simulink model "RW_1"  (R2018a)
settings: Solver=ode4  StartTime=0  StopTime=25000  FixedStep=ConfParam.confOrbit.dt  RelTol=1e-3
undefined symbols (not defined in the file): ConfParam
libraries: sharedtransform x2, Command x1, Date x1, KepOrbit x1, Estimator x1, BdotController x1, RWS_PDcontroller x1, IGRF x1, SunEphemeris_MathWorks x1, MTB x1, Magnetometer x1, AeroTorqueA x1
settings Model: Creator=Cédric  LastModifiedBy=Cédric
settings DataIOCC: SaveTime=off
settings DebuggingCC: MultiTaskRateTransMsg=warning

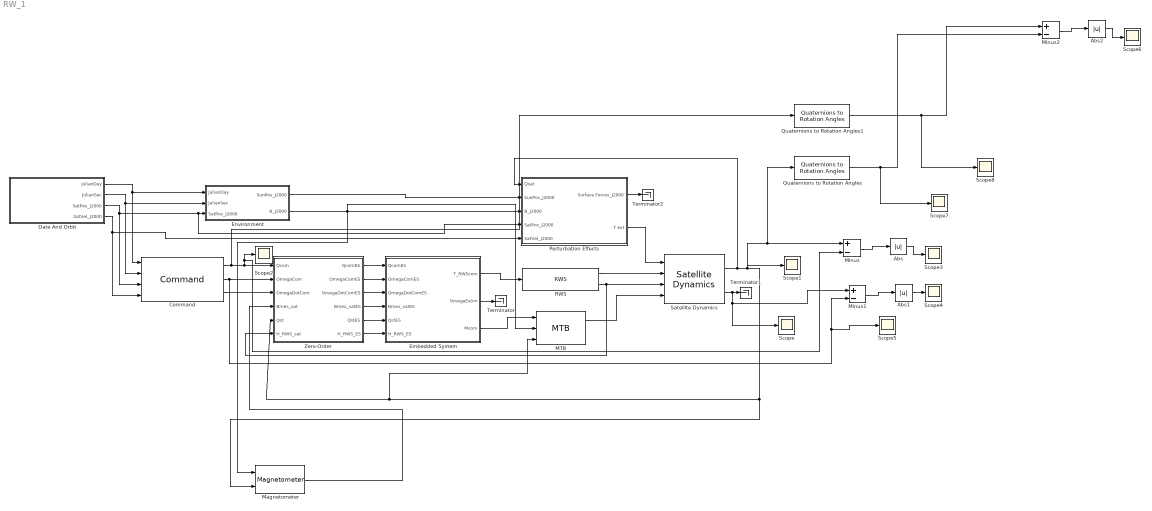
== system RW_1 ==
  Abs : Abs
  Abs1 : Abs
  Abs2 : Abs
  Command : Command/Command
  Date And Orbit : Subsystem
  Embedded System : Subsystem
  Environment : Subsystem
  MTB : MTB/MTB
  Magnetometer : Magnetometer/Magnetometer
  Minus : Sum  Inputs=+-
  Minus1 : Sum  Inputs=+-
  Minus2 : Sum  Inputs=+-
  Perturbation Effects : Subsystem
  Quaternions to Rotation Angles : sharedtransform/Quaternions to Rotation Angles  rotationOrder=ZYX  aMode=aMode
      settings: SourceProductBaseCode=AE
  Quaternions to Rotation Angles1 : sharedtransform/Quaternions to Rotation Angles  rotationOrder=ZYX  aMode=aMode
      settings: SourceProductBaseCode=AE
  RWS : RWS/RWS
  Satellite Dynamics : SatDyn/Satellite Dynamics
  Scope{,1..8} (9 alike) : Scope
  Terminator : Terminator
  Terminator1 : Terminator
  Terminator2 : Terminator
  Zero-Order : Subsystem
  wires:
  Date And Orbit/1(JulianDay) -> Environment/1(JulianDay), Command/1
  Date And Orbit/2(JulianSec) -> Environment/2(JulianSec), Command/2
  Date And Orbit/3(SatPos_J2000) -> Perturbation Effects/4(SatPos_J2000), Environment/3(SatPos_J2000), Command/3
  Date And Orbit/4(SatVel_J2000) -> Perturbation Effects/5(SatVel_J2000), Command/4
  Environment/1(SunPos_J2000) -> Perturbation Effects/2(SunPos_J2000)
  Environment/2(B_J2000) -> Perturbation Effects/3(B_J2000), Magnetometer/1, MTB/2
  Command/1 -> Quaternions to Rotation Angles1/1, Minus/2, Scope2/1, Zero-Order/1(Qcom)
  Command/2 -> Scope5/1, Minus1/2, Zero-Order/2(OmegaCom)
  Command/3 -> Zero-Order/3(OmegaDotCom)
  Zero-Order/1(QcomES) -> Embedded System/1(QcomES)
  Zero-Order/2(OmegaComES) -> Embedded System/2(OmegaComES)
  Zero-Order/3(OmegaDotComES) -> Embedded System/3(OmegaDotComES)
  Zero-Order/4(Bmes_satES) -> Embedded System/4(Bmes_satES)
  Zero-Order/5(QstES) -> Embedded System/5(QstES)
  Zero-Order/6(H_RWS_ES) -> Embedded System/6(H_RWS_ES)
  Embedded System/1(T_RWScom) -> RWS/1
  Embedded System/3(Mcom) -> MTB/1
  Satellite Dynamics/1 -> Perturbation Effects/1(Qsat), Scope1/1, Quaternions to Rotation Angles/1, Minus/1, MTB/3, Zero-Order/5(Qst), Magnetometer/2
  RWS/2 -> Satellite Dynamics/3, Zero-Order/6(H_RWS_sat)
  Perturbation Effects/2(T ext) -> Satellite Dynamics/1
  RWS/1 -> Satellite Dynamics/2
  MTB/1 -> Satellite Dynamics/4
  Magnetometer/1 -> Zero-Order/4(Bmes_sat)
  Embedded System/2(OmegaEstim) -> Terminator/1
  Satellite Dynamics/2 -> Minus1/1, Scope/1, Terminator1/1
  Perturbation Effects/1(Surface Forces_J2000) -> Terminator2/1
  Minus/1 -> Abs/1
  Abs/1 -> Scope3/1
  Minus1/1 -> Abs1/1
  Abs1/1 -> Scope4/1
  Abs2/1 -> Scope6/1
  Minus2/1 -> Abs2/1
  Quaternions to Rotation Angles1/1 -> Scope8/1, Minus2/1
  Quaternions to Rotation Angles/1 -> Scope7/1, Minus2/2

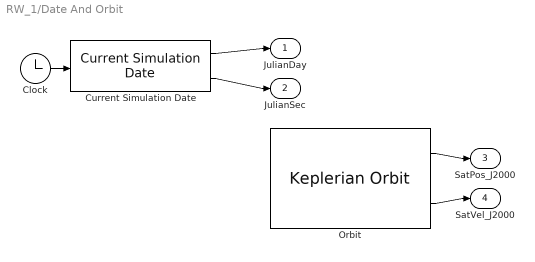
== system RW_1/Date And Orbit ==
  Clock : Clock
  Current Simulation Date : Date/Current Simulation Date
  Orbit : KepOrbit/Keplerian Orbit
  JulianDay : Outport
  JulianSec : Outport  Port=2
  SatPos_J2000 : Outport  Port=3
  SatVel_J2000 : Outport  Port=4
  wires:
  Current Simulation Date/1 -> JulianDay/1
  Current Simulation Date/2 -> JulianSec/1
  Clock/1 -> Current Simulation Date/1
  Orbit/1 -> SatPos_J2000/1
  Orbit/2 -> SatVel_J2000/1

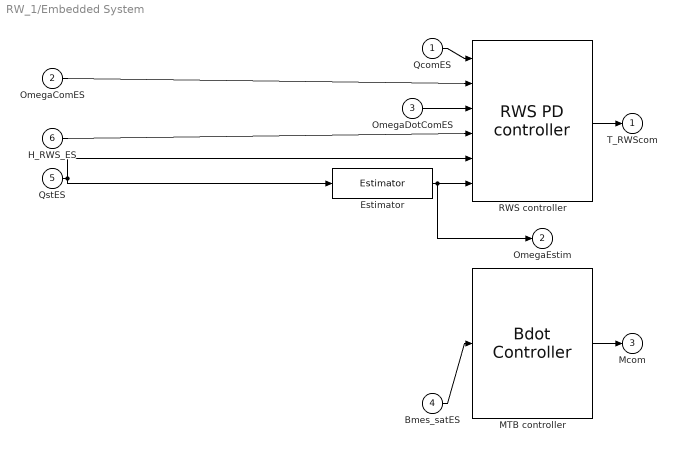
== system RW_1/Embedded System ==
  QcomES : Inport
  OmegaComES : Inport  Port=2
  OmegaDotComES : Inport  Port=3
  Bmes_satES : Inport  Port=4
  QstES : Inport  Port=5
  H_RWS_ES : Inport  Port=6
  Estimator : Estimator/Estimator
  MTB controller : BdotController/Bdot Controller
  RWS controller : RWS_PDcontroller/RWS PD controller
  T_RWScom : Outport
  OmegaEstim : Outport  Port=2
  Mcom : Outport  Port=3
  wires:
  QcomES/1 -> RWS controller/1
  OmegaComES/1 -> RWS controller/2
  OmegaDotComES/1 -> RWS controller/3
  H_RWS_ES/1 -> RWS controller/4
  QstES/1 -> RWS controller/5, Estimator/1
  Estimator/1 -> RWS controller/6, OmegaEstim/1
  RWS controller/1 -> T_RWScom/1
  Bmes_satES/1 -> MTB controller/1
  MTB controller/1 -> Mcom/1

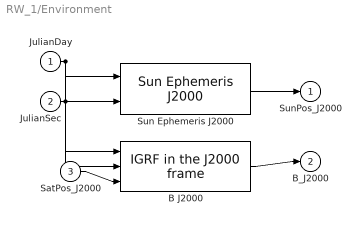
== system RW_1/Environment ==
  JulianDay : Inport
  JulianSec : Inport  Port=2
  SatPos_J2000 : Inport  Port=3
  B J2000 : IGRF/IGRF in the J2000 frame
  Sun Ephemeris J2000 : SunEphemeris_MathWorks/Sun Ephemeris J2000
  SunPos_J2000 : Outport
  B_J2000 : Outport  Port=2
  wires:
  Sun Ephemeris J2000/1 -> SunPos_J2000/1
  JulianDay/1 -> Sun Ephemeris J2000/1, B J2000/1
  JulianSec/1 -> Sun Ephemeris J2000/2, B J2000/2
  SatPos_J2000/1 -> B J2000/3
  B J2000/1 -> B_J2000/1

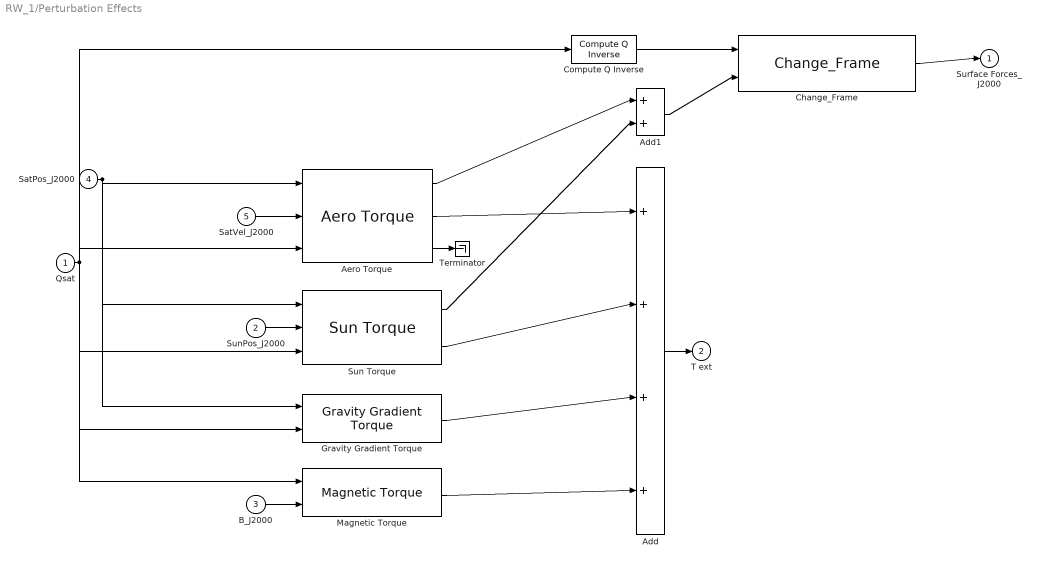
== system RW_1/Perturbation Effects ==
  Qsat : Inport
  SunPos_J2000 : Inport  Port=2
  B_J2000 : Inport  Port=3
  SatPos_J2000 : Inport  Port=4
  SatVel_J2000 : Inport  Port=5
  Add : Sum  Inputs=++++
  Add1 : Sum
  Aero Torque : AeroTorqueA/Aero Torque
  Change_Frame : ChangeFrame/Change_Frame
  Compute Q Inverse : Qinverse/Compute Q Inverse
  Gravity Gradient Torque : GravGradTorque/Gravity Gradient Torque
  Magnetic Torque : MagnTorque/Magnetic Torque
  Sun Torque : SunTorqueA/Sun Torque
  Terminator : Terminator
  Surface Forces_J2000 : Outport
  T ext : Outport  Port=2
  wires:
  Compute Q Inverse/1 -> Change_Frame/1
  Change_Frame/1 -> Surface Forces_J2000/1
  Qsat/1 -> Compute Q Inverse/1, Gravity Gradient Torque/2, Sun Torque/3, Magnetic Torque/1, Aero Torque/3
  SunPos_J2000/1 -> Sun Torque/2
  B_J2000/1 -> Magnetic Torque/2
  SatPos_J2000/1 -> Sun Torque/1, Gravity Gradient Torque/1, Aero Torque/1
  SatVel_J2000/1 -> Aero Torque/2
  Aero Torque/3 -> Terminator/1
  Add1/1 -> Change_Frame/2
  Aero Torque/1 -> Add1/1
  Sun Torque/1 -> Add1/2
  Add/1 -> T ext/1
  Aero Torque/2 -> Add/1
  Sun Torque/2 -> Add/2
  Gravity Gradient Torque/1 -> Add/3
  Magnetic Torque/1 -> Add/4

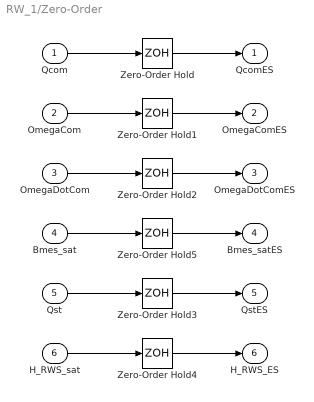
== system RW_1/Zero-Order ==
  Qcom : Inport
  OmegaCom : Inport  Port=2
  OmegaDotCom : Inport  Port=3
  Bmes_sat : Inport  Port=4
  Qst : Inport  Port=5
  H_RWS_sat : Inport  Port=6
  Zero-Order Hold{,1..5} (6 alike) : ZeroOrderHold  SampleTime=1/ConfParam.confES.frequency
  QcomES : Outport
  OmegaComES : Outport  Port=2
  OmegaDotComES : Outport  Port=3
  Bmes_satES : Outport  Port=4
  QstES : Outport  Port=5
  H_RWS_ES : Outport  Port=6
  wires:
  Qcom/1 -> Zero-Order Hold/1
  Zero-Order Hold/1 -> QcomES/1
  OmegaCom/1 -> Zero-Order Hold1/1
  Zero-Order Hold1/1 -> OmegaComES/1
  OmegaDotCom/1 -> Zero-Order Hold2/1
  Zero-Order Hold2/1 -> OmegaDotComES/1
  Qst/1 -> Zero-Order Hold3/1
  Zero-Order Hold3/1 -> QstES/1
  H_RWS_sat/1 -> Zero-Order Hold4/1
  Zero-Order Hold4/1 -> H_RWS_ES/1
  Bmes_sat/1 -> Zero-Order Hold5/1
  Zero-Order Hold5/1 -> Bmes_satES/1
